simulink model "JointSpaceControl_own_MCP"  (R2013a)
settings: Solver=ode45  StartTime=0.0  StopTime=sim_end  MaxStep=0.008  RelTol=1e-3
PreLoadFcn:
  | Initialization
InitFcn:
  | Initialization
values from neighbouring files (symbols this model uses):
  a_max = [27 27 27 27 27 27]    [Initialization.m]
  dq_0 = qd_actual.signals.values(1,:)    [Initialization.m]
  K_0 = [            omega_1, zeros(1,5);         0,          omega_2, zeros(1,4);         zeros(1,2), omega_3, zeros(1,3);         zeros(1,3), omega_4, zeros(1,2);         zeros(1,4), omega_5, 0;         zeros(1,5), omega_6]    [Initialization.m]
  K_1 = [            omega_7, zeros(1,5);         0,          omega_8, zeros(1,4);         zeros(1,2), omega_9, zeros(1,3);         zeros(1,3), omega_10, zeros(1,2);         zeros(1,4), omega_11, 0;         zeros(1,5), omega_12]    [Initialization.m]
  q_0 = q_actual.signals.values(1,:)    [Initialization.m]
  q_max = 2*pi*ones(1,6)    [Initialization.m]
  q_min = -2*pi*ones(1,6)    [Initialization.m]
  torque_max = [150 150 150 28 28 28]    [Initialization.m]
  v_max = 3.4*ones(1,6)    [Initialization.m]
(part 4 of 4)

== matlab function JointSpaceControl_own_MCP/Forward & Velocity Kinematics Joint -> Tool Geometric Jacobian/base_tool_transformation_matrix ==
  data: d output; q input; R output
function [d, R]   = base_tool_transformation(q)
% BASE_TOOL_TRANSFORMATION - Transformationmatrix from Base to Tool.
%  Calculates the Base-Tool Transformation matrix based on the current
%  joint positions and returns the rotation matrix and the displacement
%  vector.

theta1 = q(1);
theta2 = q(2);
theta3 = q(3);
theta4 = q(4);
theta5 = q(5);
theta6 = q(6);

T = [(((cos(theta1) * cos(theta2) * cos(theta3) - cos(theta1) * sin(theta2) ...
    * sin(theta3)) * cos(theta4) + (-cos(theta1) * cos(theta2) * sin(theta3) ...
    - cos(theta1) * sin(theta2) * cos(theta3)) * sin(theta4)) * cos(theta5) ...
    + sin(theta1) * sin(theta5)) * cos(theta6) + (-(cos(theta1) * cos(theta2) ...
    * cos(theta3) - cos(theta1) * sin(theta2) * sin(theta3)) * sin(theta4) + ...
    (-cos(theta1) * cos(theta2) * sin(theta3) - cos(theta1) * sin(theta2) * ...
    cos(theta3)) * cos(theta4)) * sin(theta6) -(((cos(theta1) * cos(theta2) * ...
    cos(theta3) - cos(theta1) * sin(theta2) * sin(theta3)) * cos(theta4) + ...
    (-cos(theta1) * cos(theta2) * sin(theta3) - cos(theta1) * sin(theta2) * ...
    cos(theta3)) * sin(theta4)) * cos(theta5) + sin(theta1) * sin(theta5)) * ...
    sin(theta6) + (-(cos(theta1) * cos(theta2) * cos(theta3) - cos(theta1) * ...
    sin(theta2) * sin(theta3)) * sin(theta4) + (-cos(theta1) * cos(theta2) * ...
    sin(theta3) - cos(theta1) * sin(theta2) * cos(theta3)) * cos(theta4)) * ...
    cos(theta6) -((cos(theta1) * cos(theta2) * cos(theta3) - cos(theta1) * ...
    sin(theta2) * sin(theta3)) * cos(theta4) + (-cos(theta1) * cos(theta2) * ...
    sin(theta3) - cos(theta1) * sin(theta2) * cos(theta3)) * sin(theta4)) * ...
    sin(theta5) + sin(theta1) * cos(theta5) -0.082 * ((cos(theta1) * ...
    cos(theta2) * cos(theta3) - cos(theta1) * sin(theta2) * sin(theta3)) * ...
    cos(theta4) + (-cos(theta1) * cos(theta2) * sin(theta3) - cos(theta1) * ...
    sin(theta2) * cos(theta3)) * sin(theta4)) * sin(theta5) + 0.082 * ...
    sin(theta1) * cos(theta5) + 0.093 * (cos(theta1) * cos(theta2) * ...
    cos(theta3) - cos(theta1) * sin(theta2) * sin(theta3)) * sin(theta4) - ...
    0.093 * (-cos(theta1) * cos(theta2) * sin(theta3) - cos(theta1) * ...
    sin(theta2) * cos(theta3)) * cos(theta4) + 0.109 * sin(theta1) - ...
    0.39243 * cos(theta1) * cos(theta2) * cos(theta3) + 0.39243 * ...
    cos(theta1) * sin(theta2) * sin(theta3) - 0.425 * cos(theta1) * cos(theta2); ...
    (((sin(theta1) * cos(theta2) * cos(theta3) - sin(theta1) * sin(theta2) * ...
    sin(theta3)) * cos(theta4) + (-sin(theta1) * cos(theta2) * sin(theta3) - ...
    sin(theta1) * sin(theta2) * cos(theta3)) * sin(theta4)) * cos(theta5) - ...
    cos(theta1) * sin(theta5)) * cos(theta6) + (-(sin(theta1) * cos(theta2) * ...
    cos(theta3) - sin(theta1) * sin(theta2) * sin(theta3)) * sin(theta4) + ...
    (-sin(theta1) * cos(theta2) * sin(theta3) - sin(theta1) * sin(theta2) * ...
    cos(theta3)) * cos(theta4)) * sin(theta6) -(((sin(theta1) * cos(theta2) *...
    cos(theta3) - sin(theta1) * sin(theta2) * sin(theta3)) * cos(theta4) + ...
    (-sin(theta1) * cos(theta2) * sin(theta3) - sin(theta1) * sin(theta2) * ...
    cos(theta3)) * sin(theta4)) * cos(theta5) - cos(theta1) * sin(theta5)) * ...
    sin(theta6) + (-(sin(theta1) * cos(theta2) * cos(theta3) - sin(theta1) * ...
    sin(theta2) * sin(theta3)) * sin(theta4) + (-sin(theta1) * cos(theta2) * ...
    sin(theta3) - sin(theta1) * sin(theta2) * cos(theta3)) * cos(theta4)) * ...
    cos(theta6) -((sin(theta1) * cos(theta2) * cos(theta3) - sin(theta1) * ...
    sin(theta2) * sin(theta3)) * cos(theta4) + (-sin(theta1) * cos(theta2) * ...
    sin(theta3) - sin(theta1) * sin(theta2) * cos(theta3)) * sin(theta4)) *...
     sin(theta5) - cos(theta1) * cos(theta5) -0.082 * ((sin(theta1) * ...
    cos(theta2) * cos(theta3) - sin(theta1) * sin(theta2) * sin(theta3)) * ...
    cos(theta4) + (-sin(theta1) * cos(theta2) * sin(theta3) - sin(theta1) * ...
    sin(theta2) * cos(theta3)) * sin(theta4)) * sin(theta5) - 0.082 * ...
    cos(theta1) * cos(theta5) + 0.093 * (sin(theta1) * cos(theta2) * ...
    cos(theta3) - sin(theta1) * sin(theta2) * sin(theta3)) * sin(theta4) - ...
    0.093 * (-sin(theta1) * cos(theta2) * sin(theta3) - sin(theta1) * ...
    sin(theta2) * cos(theta3)) * cos(theta4) - 0.109 * cos(theta1) - ...
    0.39243 * sin(theta1) * cos(theta2) * cos(theta3) + 0.39243 * ...
    sin(theta1) * sin(theta2) * sin(theta3) - 0.425 * sin(theta1) * ...
    cos(theta2); ((sin(theta2) * cos(theta3) + cos(theta2) * sin(theta3)) ...
    * cos(theta4) + (-sin(theta2) * sin(theta3) + cos(theta2) * cos(theta3)) ...
    * sin(theta4)) * cos(theta5) * cos(theta6) + (-(sin(theta2) * cos(theta3) ...
    + cos(theta2) * sin(theta3)) * sin(theta4) + (-sin(theta2) * sin(theta3) ...
    + cos(theta2) * cos(theta3)) * cos(theta4)) * sin(theta6) -((sin(theta2) ...
    * cos(theta3) + cos(theta2) * sin(theta3)) * cos(theta4) + (-sin(theta2) ...
    * sin(theta3) + cos(theta2) * cos(theta3)) * sin(theta4)) * cos(theta5) ...
    * sin(theta6) + (-(sin(theta2) * cos(theta3) + cos(theta2) * sin(theta3)) ...
    * sin(theta4) + (-sin(theta2) * sin(theta3) + cos(theta2) * cos(theta3)) ...
    * cos(theta4)) * cos(theta6) -((sin(theta2) * cos(theta3) + cos(theta2) ...
    * sin(theta3)) * cos(theta4) + (-sin(theta2) * sin(theta3) + cos(theta2) ...
    * cos(theta3)) * sin(theta4)) * sin(theta5) 0.0892 - 0.082 * ...
    ((sin(theta2) * cos(theta3) + cos(theta2) * sin(theta3)) * cos(theta4) ...
    + (-sin(theta2) * sin(theta3) + cos(theta2) * cos(theta3)) * sin(theta4)) ...
    * sin(theta5) + 0.093 * (sin(theta2) * cos(theta3) + cos(theta2) * ...
    sin(theta3)) * sin(theta4) - 0.093 * (-sin(theta2) * sin(theta3) + ...
    cos(theta2) * cos(theta3)) * cos(theta4) - 0.39243 * sin(theta2) * ...
    cos(theta3) - 0.39243 * cos(theta2) * sin(theta3) - 0.425 * sin(theta2); ...
    0 0 0 1;];

R = T(1:3,1:3);
d = T(1:3,4);

end

== matlab function JointSpaceControl_own_MCP/Forward & Velocity Kinematics Joint -> Tool Geometric Jacobian/Euler -> R ==
  data: theta input; phi input; R output; psi input
function R   = Euler_angle_to_R(theta, phi, psi)
%R_TO_EULER_ANGLE Transform rotation matrix to euler-angle format, where
%the rotation happens around ZYZ, with R_ZYZ = R_Z,phi*R_Y,theta*R_Z,psi

r_11 = cos(phi)*cos(theta)*cos(psi)-sin(phi)*sin(psi);
r_12 = -cos(phi)*cos(theta)*sin(psi)-sin(phi)*cos(psi);
r_13 = cos(phi)*sin(theta);

r_21 = sin(phi)*cos(theta)*cos(psi) + cos(phi)*sin(psi);
r_22 = -sin(phi)*cos(theta)*sin(psi)+cos(phi)*cos(psi);
r_23 = sin(phi)*sin(theta);

r_31 = -sin(theta)*cos(psi);
r_32 = sin(theta)*sin(psi);
r_33 = cos(theta);

R = [r_11, r_12, r_13; ...
     r_21, r_22, r_23; ...
     r_31, r_32, r_33];
end

== matlab function JointSpaceControl_own_MCP/Forward & Velocity Kinematics Joint -> Tool Geometric Jacobian/Joints -> End-Effector/from_me2 ==
  data: J_a input; dJ_a input; dq input; ddq input; ddX output
function ddX     = ddX(J_a, dJ_a, dq, ddq)
% ANALYTICAL JACOBIAN - Jacobian from Base to Tool.
%  Calculates the analytical Jacobian, based on the Euler angle transform
%  representation.

ddX = J_a*ddq + dJ_a*dq;

end

== matlab function JointSpaceControl_own_MCP/Forward & Velocity Kinematics Joint -> Tool Geometric Jacobian/Joints -> End-Effector/from_me4 ==
  data: J_a input; dq input; dX output
function dX     = dX(J_a, dq)
% ANALYTICAL JACOBIAN - Jacobian from Base to Tool.
%  Calculates the analytical Jacobian, based on the Euler angle transform
%  representation.

dX = J_a*dq;

end

== matlab function JointSpaceControl_own_MCP/Forward & Velocity Kinematics Joint -> Tool Geometric Jacobian/End-Effector -> Joints/from_me5 ==
  data: J_a input; dq output; dX input
function dq     = dq(J_a, dX)
% ANALYTICAL JACOBIAN - Jacobian from Base to Tool.
%  Calculates the analytical Jacobian, based on the Euler angle transform
%  representation.

dq = inv(J_a)*dX;

end

== matlab function JointSpaceControl_own_MCP/Forward & Velocity Kinematics Joint -> Tool Geometric Jacobian/End-Effector -> Joints/from_me6 ==
  data: J_a input; dJ_a input; ddX input; dq input; ddq output
function ddq     = ddq(J_a, dJ_a, ddX, dq)
% ANALYTICAL JACOBIAN - Jacobian from Base to Tool.
%  Calculates the analytical Jacobian, based on the Euler angle transform
%  representation.

ddq = inv(J_a)*(ddX - dJ_a*dq);

end

== matlab function JointSpaceControl_own_MCP/Inverse Dynamics M, C, g1/ur5_invDynamics ==
  data: a_q input; M input; G input; CDq input; tau output
function tau = ur5_invDynamics(a_q, M, G, CDq)
%#codegen
%Returns the torque that must be applied to the robot given the desired
%position, velocity and acceleration
tau = M*a_q + CDq + G;

== matlab function JointSpaceControl_own_MCP/Robot UR5 M, C, g/ur5_dynamics ==
  data: q input; dq input; tau input; ddq output
function ddq = ur5_dynamics( q, dq, tau )
%#codegen
%Returns the acceleration of the manipulator based on its dynamics
[ M, G, CDq ] = ur5_matrices( q, dq );

ddq = M \ (tau - CDq - G);

== matlab function JointSpaceControl_own_MCP/Inverse Dynamics M, C, g/MATLAB Function ==
  data: q input; G_Angel output
function G_Angel  = UR5_G_Angel(q)
%#codegen
%Returns the dynamics of the UR5 manipulator


m2 = 8.393;
m3 = 2.275;
	G_Angel = [0 ; ...
        -0.2084625e1 * m2 * sin(q(2)) + m3 * (0.11765133e1 * sin(q(2)) * ...
        cos(q(3)) - 0.26714592e1 * cos(q(2)) * sin(q(3)) - 0.981e1 * ...
        (0.39225e0 * cos(q(3)) + 0.425e0) * sin(q(2))) ; ...
        m3 * (-0.26714592e1 * ...
        cos(q(2)) * sin(q(3)) - 0.26714592e1 * sin(q(2)) * cos(q(3)))];
end

== matlab function JointSpaceControl_own_MCP/Inverse Dynamics M, C, g/MATLAB Function1 ==
  data: q input; G_Version1 output
function G_Version1  = UR5_G_Version1(q)
%#codegen
%Returns the dynamics of the UR5 manipulator


G_Version1 = [0 ; ...
    -0.1749625762e2 * sin(q(2)) + 0.2676567758e1 * sin(q(2)) * ...
    cos(q(3)) - 0.1076824816e2 * cos(q(2)) * sin(q(3)) - 0.3427614e2 * ...
    (0.39225e0 * cos(q(3)) + 0.425e0) * sin(q(2)) + 0.1954000926e0 * ...
    (-cos(q(2)) * cos(q(3)) + sin(q(2)) * sin(q(3))) * sin(q(4)) + 0.1738749906e0 * ...
    cos(q(4)) * (-sin(q(2)) * cos(q(3)) - cos(q(2)) * sin(q(3))) + 0.21525102e-1 * ...
    sin(q(4)) * (-sin(q(2)) * sin(q(3)) + cos(q(2)) * cos(q(3))) + 0.1932637091e0 * ...
    sin(q(5)) * (sin(q(4)) * (-sin(q(2)) * cos(q(3)) - cos(q(2)) * sin(q(3))) + cos(q(4)) * ...
    (-sin(q(2)) * sin(q(3)) + cos(q(2)) * cos(q(3)))) - 0.1195839e2 * ((0.9465e-1 * ...
    cos(q(4)) + 0.39225e0) * cos(q(3)) - 0.9465e-1 * sin(q(4)) * sin(q(3)) + 0.425e0) * ...
    sin(q(2)) - 0.1131861614e1 * sin(q(4)) * cos(q(2)) * cos(q(3)) + 0.1195839e2 * ...
    (-0.9465e-1 * cos(q(4)) - 0.39225e0) * sin(q(3)) * cos(q(2)) - 0.1843299e1 * ...
    ((0.823e-1 * sin(q(5)) * sin(q(4)) + 0.9465e-1 * cos(q(4)) + 0.39225e0) * ...
    cos(q(3)) + 0.425e0 + (0.823e-1 * sin(q(5)) * cos(q(4)) - 0.9465e-1 * ...
    sin(q(4))) * sin(q(3))) * sin(q(2)) + 0.1843299e1 * (0.823e-1 * sin(q(5)) * ...
    cos(q(4)) - 0.9465e-1 * sin(q(4))) * cos(q(2)) * cos(q(3)) + 0.1843299e1 * ...
    (-0.39225e0 - 0.823e-1 * sin(q(5)) * sin(q(4)) - 0.9465e-1 * cos(q(4))) * ...
    sin(q(3)) * cos(q(2)) ; ...
    -0.1076824816e2 * cos(q(2)) * sin(q(3)) - 0.1076824816e2 * ...
    sin(q(2)) * cos(q(3)) + 0.1954000926e0 * (-cos(q(2)) * cos(q(3)) + sin(q(2)) * ...
    sin(q(3))) * sin(q(4)) + 0.1738749906e0 * cos(q(4)) * (-sin(q(2)) * ...
    cos(q(3)) - cos(q(2)) * sin(q(3))) + 0.21525102e-1 * sin(q(4)) * ...
    (-sin(q(2)) * sin(q(3)) + cos(q(2)) * cos(q(3))) + 0.1932637091e0 * ...
    sin(q(5)) * (sin(q(4)) * (-sin(q(2)) * cos(q(3)) - cos(q(2)) * ...
    sin(q(3))) + cos(q(4)) * (-sin(q(2)) * sin(q(3)) + cos(q(2)) * ...
    cos(q(3)))) + 0.1195839e2 * (-(0.9465e-1 * cos(q(4)) + 0.39225e0) * ...
    sin(q(3)) - 0.9465e-1 * sin(q(4)) * cos(q(3))) * cos(q(2)) + 0.1131861614e1 * ...
    sin(q(4)) * sin(q(2)) * sin(q(3)) + 0.1195839e2 * (-0.9465e-1 * cos(q(4)) - 0.39225e0) * ...
    cos(q(3)) * sin(q(2)) + 0.1843299e1 * (-(0.823e-1 * sin(q(5)) * sin(q(4)) + 0.9465e-1 *  ...
    cos(q(4)) + 0.39225e0) * sin(q(3)) + (0.823e-1 * sin(q(5)) * cos(q(4)) - 0.9465e-1 *  ...
    sin(q(4))) * cos(q(3))) * cos(q(2)) - 0.1843299e1 * (0.823e-1 * sin(q(5)) *  ...
    cos(q(4)) - 0.9465e-1 * sin(q(4))) * sin(q(2)) * sin(q(3)) + 0.1843299e1 *  ...
    (-0.39225e0 - 0.823e-1 * sin(q(5)) * sin(q(4)) - 0.9465e-1 * cos(q(4))) *  ...
    cos(q(3)) * sin(q(2)) ; ...
    0.1954000926e0 * cos(q(4)) * (-sin(q(2)) *  ...
    cos(q(3)) - cos(q(2)) * sin(q(3))) - 0.1738749906e0 * sin(q(4)) *  ...
    (-sin(q(2)) * sin(q(3)) + cos(q(2)) * cos(q(3))) + 0.21525102e-1 *  ...
    (cos(q(2)) * sin(q(3)) + sin(q(2)) * cos(q(3))) * cos(q(4)) + 0.1932637091e0 *  ...
    sin(q(5)) * (-(cos(q(2)) * sin(q(3)) + sin(q(2)) * cos(q(3))) *  ...
    sin(q(4)) + cos(q(4)) * (-sin(q(2)) * sin(q(3)) + cos(q(2)) *  ...
    cos(q(3)))) + 0.1195839e2 * (-0.9465e-1 * sin(q(4)) * cos(q(3)) - 0.9465e-1 *  ...
    cos(q(4)) * sin(q(3))) * cos(q(2)) - 0.1131861614e1 * cos(q(4)) *  ...
    sin(q(2)) * cos(q(3)) + 0.1131861614e1 * sin(q(4)) * sin(q(2)) *  ...
    sin(q(3)) + 0.1843299e1 * ((0.823e-1 * sin(q(5)) * cos(q(4)) - 0.9465e-1 *  ...
    sin(q(4))) * cos(q(3)) + (-0.823e-1 * sin(q(5)) * sin(q(4)) - 0.9465e-1 *  ...
    cos(q(4))) * sin(q(3))) * cos(q(2)) + 0.1843299e1 * (-0.823e-1 * sin(q(5)) *  ...
    sin(q(4)) - 0.9465e-1 * cos(q(4))) * sin(q(2)) * cos(q(3)) + 0.1843299e1 *  ...
    (-0.823e-1 * sin(q(5)) * cos(q(4)) + 0.9465e-1 * sin(q(4))) * sin(q(3)) *  ...
    sin(q(2)) ; ...
    0.1932637091e0 * ((cos(q(2)) * sin(q(3)) + sin(q(2)) * cos(q(3))) *  ...
    cos(q(4)) + sin(q(4)) * (-sin(q(2)) * sin(q(3)) + cos(q(2)) * cos(q(3)))) *  ...
    cos(q(5)) + 0.1843299e1 * (0.823e-1 * cos(q(5)) * sin(q(4)) *  ...
    cos(q(3)) + 0.823e-1 * cos(q(5)) * cos(q(4)) * sin(q(3))) *  ...
    cos(q(2)) + 0.1517035077e0 * cos(q(5)) * cos(q(4)) * sin(q(2)) *  ...
    cos(q(3)) - 0.1517035077e0 * cos(q(5)) * sin(q(4)) * sin(q(3)) * sin(q(2)) ; ...
    0];
end

== matlab function JointSpaceControl_own_MCP/Inverse Dynamics M, C, g/MATLAB Function6 ==
  data: a_q input; M input; G input; CDq input; tau output; tau_M output; tau_CDq output; tau_G output
function [tau, tau_M, tau_CDq, tau_G] = ur5_invDynamics(a_q, M, G, CDq)
%#codegen
%Returns the torque that must be applied to the robot given the desired
%position, velocity and acceleration
tau = M*a_q + CDq + G;
tau_M = M*a_q;
tau_CDq = CDq;
tau_G = G;
